simulink model "Encoder_compensado"  (R2015a)
settings: Solver=ode45  StartTime=0.0  StopTime=800  RelTol=1e-3
undefined symbols (not defined in the file): Bm, Ga, Jt, Kb, Ki, L, PosInicial, R, RelacionEngranajes, Rrueda
libraries: cstblocks x3, simulink x1
settings Model: Creator=familia colazo  LastModifiedBy=familia colazo

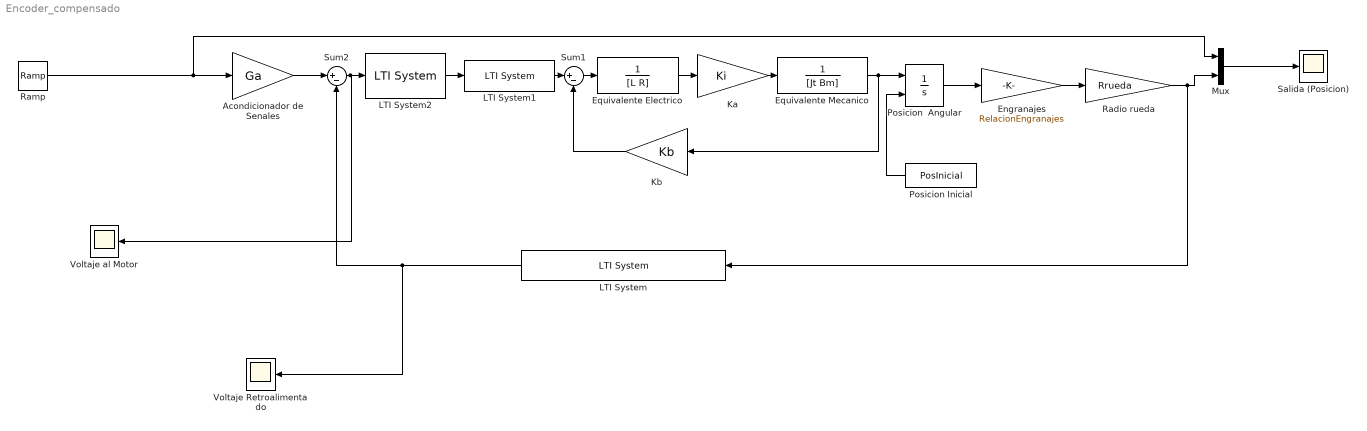
== system Encoder_compensado ==
  "Acondicionador de Senales " : Gain  Gain=Ga
  "Engranajes " : Gain  Gain=RelacionEngranajes
  Equivalente Electrico : TransferFcn  Denominator=[L R]
  Equivalente Mecanico : TransferFcn  Denominator=[Jt Bm]
  Ka : Gain  Gain=Ki
  Kb : Gain  Gain=Kb
  LTI System : cstblocks/LTI System  sys=Sensor  IC=[]
  LTI System1 : cstblocks/LTI System  sys=Comp  IC=[]
  LTI System2 : cstblocks/LTI System  sys=CompensadorAtraso  IC=[]
  Mux : Mux  Inputs=2
  Posicion  Angular : Integrator  InitialConditionSource=external
  Posicion Inicial : Constant  Value=PosInicial
  Radio rueda : Gain  Gain=Rrueda
  Ramp : simulink/Sources/Ramp  slope=1  start=0  X0=0
  Salida (Posicion) : Scope
      settings: TickLabels=on  TimeRange=14  YMin=483  YMax=497  SampleInput=on
  Sum1 : Sum  Inputs=|+-
  Sum2 : Sum  Inputs=|+-
  Voltaje Retroalimentado : Scope
      settings: TickLabels=on  TimeRange=14  YMin=-0.751036  YMax=0.0612263  SampleInput=on
  Voltaje al Motor : Scope
      settings: TickLabels=on  TimeRange=14  YMin=-0.751036  YMax=0.0612263  SaveName=ScopeData2  SampleInput=on
  wires:
  Mux/1 -> Salida (Posicion)/1
  LTI System/1 -> Voltaje Retroalimentado/1, Sum2/2
  Posicion Inicial/1 -> Posicion  Angular/2
  Kb/1 -> Sum1/2
  Equivalente Mecanico/1 -> Kb/1, Posicion  Angular/1
  Equivalente Electrico/1 -> Ka/1
  Sum1/1 -> Equivalente Electrico/1
  Ka/1 -> Equivalente Mecanico/1
  "Engranajes "/1 -> Radio rueda/1
  Radio rueda/1 -> LTI System/1, Mux/2
  Posicion  Angular/1 -> "Engranajes "/1
  LTI System1/1 -> Sum1/1
  Sum2/1 -> Voltaje al Motor/1, LTI System2/1
  LTI System2/1 -> LTI System1/1
  "Acondicionador de Senales "/1 -> Sum2/1
  Ramp/1 -> Mux/1, "Acondicionador de Senales "/1
